simulink model "B2Simulink"  (R2018a)
settings: Solver=VariableStepAuto  StartTime=0.0  StopTime=300  RelTol=1e-3
libraries: dspsrcs4 x1, modelsimlib x1
settings Model: Creator=garimar  LastModifiedBy=garimar

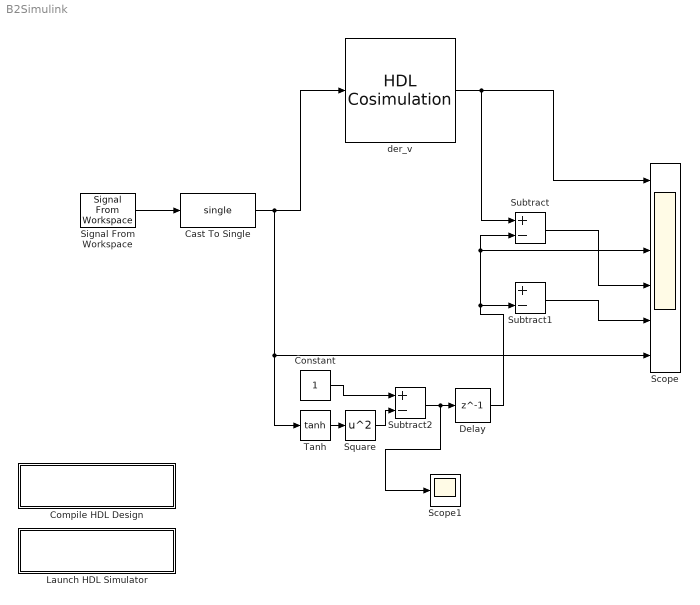
== system B2Simulink ==
  Cast To Single : DataTypeConversion  OutDataTypeStr=single
  Compile HDL Design : Subsystem
      settings: OpenFcn=eval('compile_hdl_design_der_v');
      mask Display: disp(['Double-Click to' char(10) 'compile HDL files'])
  Constant : Constant
  Delay : Delay  DelayLength=1  InitialCondition=0
  Launch HDL Simulator : Subsystem
      settings: OpenFcn=eval('launch_hdl_simulator_der_v');
      mask Display: disp(['Double-Click to' char(10) 'launch HDL simulator'])
  Scope : Scope  NumInputPorts=6
  Scope1 : Scope
  Signal From Workspace : dspsrcs4/Signal From Workspace  X=-15:0.1:15  Ts=1  nsamps=1  OutputAfterFinalValue=Setting to zero  ignoreOrWarnInputAndFrameLengths=off  OutputFrames=off
  Square : Math  Operator=square  SaturateOnIntegerOverflow=on
  Subtract : Sum  Inputs=+-
  Subtract1 : Sum  Inputs=+-
  Subtract2 : Sum  Inputs=+-
  Tanh : Trigonometry  Operator=tanh
  der_v : modelsimlib/HDL Cosimulation  PortPaths=/der_v/num_entrada;/der_v/num_salida1;  PortModes=[1 2 ]  PortTimes=[-1,1]  PortSigns=[-1,3,]  PortFracLengths=[0,0]  CommLocal=on  CommSharedMemory=off  CommPortNumber=55586  CommShowInfo=on  ClockModes=[]  ClockTimes=[]  TclPreSimCommand=force /der_v/clk 0 0 ns, 1 10 ns -repeat 20 ns;  TclPostSimCommand=|  TimingMode=ns  TimingScaleFactor=20  idxCellArray={'UNUSED_VAR'}  CosimBypass=Full Simulation  AllowDirectFeedthrough=on  ProductName=EDA Simulator Link MQ  RunAutoTimescale=off  HdlClocks=/der_v/clk 20 ns;  PreRunTime=0  PreRunTimeUnit=ns
      | noforce /der_v/clk;
      | puts "done";
      settings: SourceProductName=HDL Verifier  SourceProductBaseCode=ES
  wires:
  Signal From Workspace/1 -> Cast To Single/1
  Cast To Single/1 -> Tanh/1, Scope/6, der_v/1
  der_v/1 -> Scope/1, Subtract/1
  Subtract/1 -> Scope/4
  ? -> Subtract1/1
  Subtract1/1 -> Scope/5
  Delay/1 -> Scope/3, Subtract/2, Subtract1/2
  Subtract2/1 -> Scope1/1, Delay/1
  Constant/1 -> Subtract2/1
  Tanh/1 -> Square/1
  Square/1 -> Subtract2/2

== system B2Simulink/Compile HDL Design ==

== system B2Simulink/Launch HDL Simulator ==
